simulink model "filter"  (R2018b)
settings: Solver=VariableStepAuto  StartTime=0.0  StopTime=0.12  RelTol=1e-3
libraries: dsparch4 x4
settings Model: Creator=yangq  LastModifiedBy=yangq

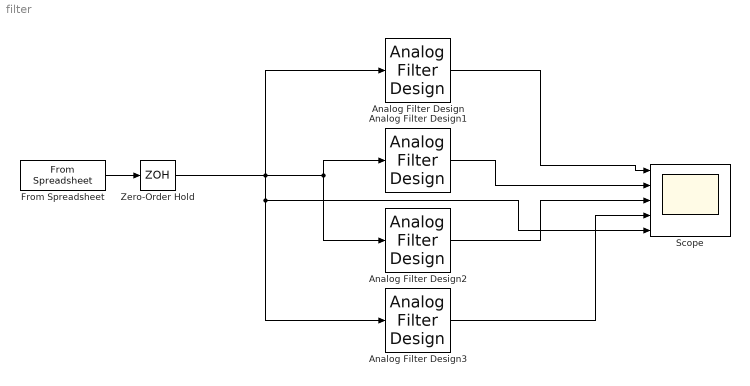
== system filter ==
  Analog Filter Design : dsparch4/Analog Filter Design  method=Butterworth  filttype=Bandpass  N=6  Wlo=2*pi*(1e06-1e05)  Whi=2*pi*(1e06+1e05)  Rp=2  Rs=40
  Analog Filter Design1 : dsparch4/Analog Filter Design  method=Chebyshev I  filttype=Bandpass  N=6  Wlo=2*pi*(1e06-1e05)  Whi=2*pi*(1e06+1e05)  Rp=2  Rs=40
  Analog Filter Design2 : dsparch4/Analog Filter Design  method=Chebyshev II  filttype=Bandpass  N=6  Wlo=2*pi*(1e06-1e05)  Whi=2*pi*(1e06+1e05)  Rp=2  Rs=40
  Analog Filter Design3 : dsparch4/Analog Filter Design  method=Elliptic  filttype=Bandpass  N=6  Wlo=2*pi*(1e06-1e05)  Whi=2*pi*(1e06+1e05)  Rp=2  Rs=40
  From Spreadsheet : FromSpreadsheet  FileName=audio.xlsx  TreatFirstColumnAs=Data  SampleTime=1/44100
  Scope : Scope  NumInputPorts=5
  Zero-Order Hold : ZeroOrderHold  SampleTime=1/44100
  wires:
  From Spreadsheet/1 -> Zero-Order Hold/1
  Analog Filter Design1/1 -> Scope/2
  Analog Filter Design2/1 -> Scope/3
  Zero-Order Hold/1 -> Analog Filter Design3/1, Scope/5, Analog Filter Design/1, Analog Filter Design2/1, Analog Filter Design1/1
  Analog Filter Design/1 -> Scope/1
  Analog Filter Design3/1 -> Scope/4
